simulink model "RBNN_Nonlinear_system_3layer_stochastic"  (R2019a)
settings: Solver=VariableStepAuto  StartTime=0.0  StopTime=inf  FixedStep=0.001  RelTol=1e-3
libraries: simulink x1
(part 1 of 3)
settings Model: NumberOfSteps=16  Creator=vardhah  LastModifiedBy=vardhah
settings DataIOCC: ReturnWorkspaceOutputs=off
settings DebuggingCC: UnderSpecifiedDimensionMsg=warning  ArithmeticOperatorsInVariantConditions=warning

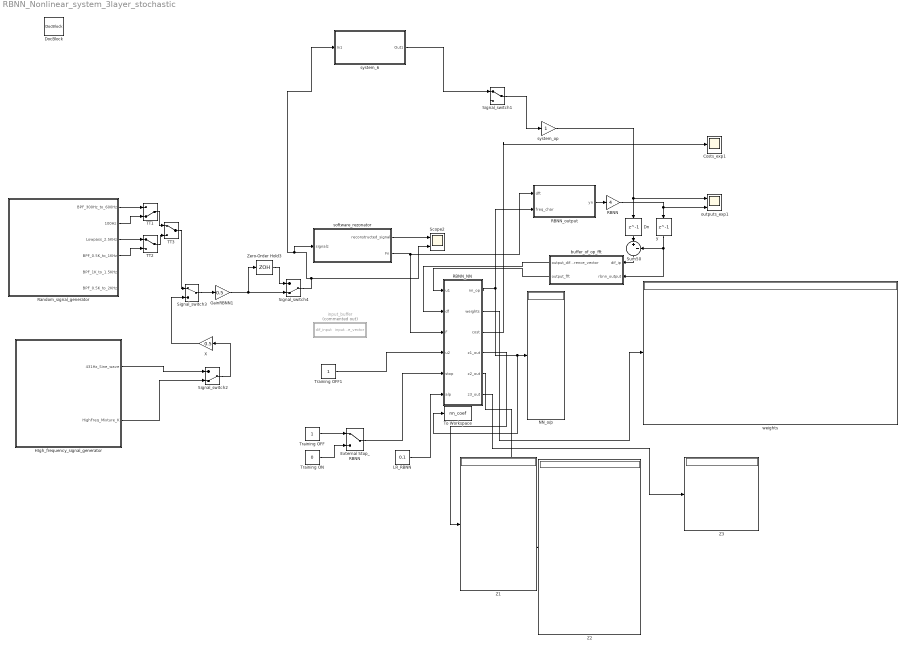
== system RBNN_Nonlinear_system_3layer_stochastic ==
  Costs_exp1 : Scope
  Dn : Delay  DelayLength=1  InitialCondition=0
  DocBlock : simulink/Model-Wide Utilities/DocBlock  DocumentType=Text
      content=|
      | system 6: gain = 0.4
      |
      | system 1b : gain= 0.2
      |
      | system 3: gain = 0.5 => cannot learn by this setup
      |
      | Training signal 373+498 rads/ s ( amplitude 0.5)
      |
      | Testing signal 1098+1431 rad/s (amplitude 0.5)
  External Stop_RBNN : ManualSwitch
  GainRBNN1 : Gain  Gain=0.5
  HIgh_frequency_signal_generator : Subsystem
  LR_RBNN : Constant  Value=0.1
  NN_o/p : Display
  RBNN : Gain  Gain=4
  RBNN_NN : MATLAB Function  TreatAsAtomicUnit=on  SystemSampleTime=0.000001
  RBNN_output : MATLAB Function  TreatAsAtomicUnit=on
  Random_signal_generator : Subsystem
  Scope2 : Scope  NumInputPorts=2
  Signal_switch1 : ManualSwitch
  Signal_switch2 : ManualSwitch  CurrentSetting=0
  Signal_switch3 : ManualSwitch
  Signal_switch4 : ManualSwitch  CurrentSetting=0
  Sum50 : Sum  Inputs=|+-
  TT1 : ManualSwitch  CurrentSetting=0
  TT2 : ManualSwitch
  TT3 : ManualSwitch
  To Workspace : ToWorkspace  VariableName=nn_coef  SaveFormat=Timeseries  SampleTime=-1
  Training OFF : Constant
  Training OFF1 : Constant
  Training ON : Constant  Value=0
  X : Gain  Gain=0.5
  Z1 : Display
  Z2 : Display
  Z3 : Display
  Zero-Order Hold3 : ZeroOrderHold  SampleTime=0.00001
  buffer_of_op_fft : MATLAB Function  TreatAsAtomicUnit=on
  input_buffer : MATLAB Function  Commented=on  TreatAsAtomicUnit=on
  outputs_exp1 : Scope  NumInputPorts=2
  software_rezonator : MATLAB Function  TreatAsAtomicUnit=on  SystemSampleTime=0.000001
  system_6 : Subsystem  TreatAsAtomicUnit=on  SystemSampleTime=0.000001
  system_op : Gain
  weights : Display
  y : Delay  DelayLength=1  InitialCondition=0
  wires:
  software_rezonator/1(reconstructed_signal) -> Scope2/1
  software_rezonator/2(Fn) -> RBNN_NN/3(F), RBNN_output/1(dft)
  RBNN_output/1(yn) -> RBNN/1
  Dn/1 -> Sum50/1
  y/1 -> buffer_of_op_fft/2(rbnn_output), Sum50/2
  RBNN_NN/1(nn_op) -> To Workspace/1, NN_o/p/1, RBNN_output/2(freq_char)
  External Stop_RBNN/1 -> RBNN_NN/5(stop)
  Training OFF/1 -> External Stop_RBNN/1
  Training ON/1 -> External Stop_RBNN/2
  RBNN_NN/3(cost) -> Costs_exp1/1
  RBNN_NN/2(weights) -> weights/1
  RBNN_NN/4(z1_out) -> Z1/1
  Sum50/1 -> buffer_of_op_fft/1(dif_ip)
  buffer_of_op_fft/1(output_difference_vector) -> RBNN_NN/2(df)
  buffer_of_op_fft/2(output_fft) -> RBNN_NN/1(u1)
  GainRBNN1/1 -> Zero-Order Hold3/1, Signal_switch4/2
  LR_RBNN/1 -> RBNN_NN/6(alp)
  Zero-Order Hold3/1 -> Signal_switch4/1
  Signal_switch4/1 -> Scope2/2, software_rezonator/1(signalz), system_6/1(In1)
  Signal_switch1/1 -> system_op/1
  system_op/1 -> outputs_exp1/1, Dn/1
  Training OFF1/1 -> RBNN_NN/4(u2)
  RBNN_NN/5(z2_out) -> Z2/1
  RBNN_NN/6(z3_out) -> Z3/1
  RBNN/1 -> outputs_exp1/2, y/1
  system_6/1(Out1) -> Signal_switch1/1
  Random_signal_generator/1(BPF_300Hz_to_600Hz) -> TT1/1
  Random_signal_generator/2(100Hz) -> TT1/2
  Random_signal_generator/3(Lowpass_2.5KHz) -> TT2/1
  Random_signal_generator/4(BPF_0.5K_to_1KHz) -> TT2/2
  TT1/1 -> TT3/1
  TT2/1 -> TT3/2
  HIgh_frequency_signal_generator/1(431Hz_Sine_wave) -> Signal_switch2/1
  HIgh_frequency_signal_generator/2(HighFreq_Mixture_K) -> Signal_switch2/2
  Signal_switch2/1 -> X/1
  Signal_switch3/1 -> GainRBNN1/1
  TT3/1 -> Signal_switch3/1
  X/1 -> Signal_switch3/2

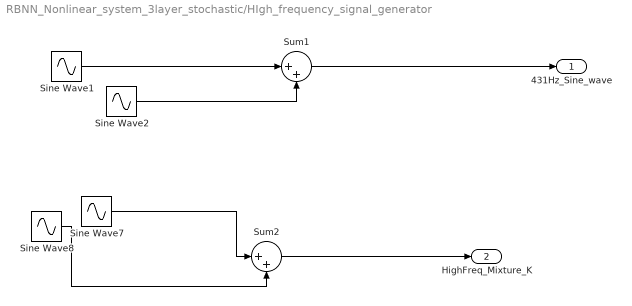
== system RBNN_Nonlinear_system_3layer_stochastic/HIgh_frequency_signal_generator ==
  Sine Wave1 : Sin  Amplitude=0.25  Frequency=1731  SampleTime=0
  Sine Wave2 : Sin  Amplitude=0.25  Frequency=1490  SampleTime=0
  Sine Wave7 : Sin  Amplitude=0.4  Frequency=2837  SampleTime=0
  Sine Wave8 : Sin  Amplitude=0.4  Frequency=2567  SampleTime=0
  Sum1 : Sum  Inputs=|++
  Sum2 : Sum  Inputs=|++
  431Hz_Sine_wave : Outport
  HighFreq_Mixture_K : Outport  Port=2
  wires:
  Sine Wave7/1 -> Sum2/1
  Sine Wave8/1 -> Sum2/2
  Sum2/1 -> HighFreq_Mixture_K/1
  Sine Wave1/1 -> Sum1/1
  Sine Wave2/1 -> Sum1/2
  Sum1/1 -> 431Hz_Sine_wave/1
